simulink model "Mixer"  (R2015a)
settings: Solver=ode2  StartTime=0.0  StopTime=10.0  FixedStep=0.01  RelTol=1e-3
InitFcn:
  | TiltCopter_Parameters_TOSTO_v3
undefined symbols (not defined in the file): Kinv, x1
settings Model: Creator=pela  LastModifiedBy=Claudio
settings HardwareCC: ProdLargestAtomicInteger=Long  ProdLargestAtomicFloat=Double  ProdEndianess=LittleEndian  ProdHWDeviceType=ARM Compatible->ARM Cortex
settings RTWCC: GenCodeOnly=on  GenerateReport=on  Toolchain=Microsoft Visual C++ 2013 v12.0 | nmake (64-bit Windows)  BuildConfiguration=Faster Runs  LaunchReport=on  TargetLang=C++
settings GRTTargetCC: MatFileLogging=off  MultiInstanceERTCode=on  CodeInterfacePackaging=C++ class

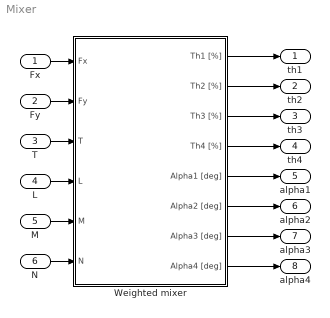
== system Mixer ==
  Fx : Inport
  Fy : Inport  Port=2
  T : Inport  Port=3
  L : Inport  Port=4
  M : Inport  Port=5
  N : Inport  Port=6
  Weighted mixer : Subsystem
  th1 : Outport
  th2 : Outport  Port=2
  th3 : Outport  Port=3
  "th4 " : Outport  Port=4
  alpha1 : Outport  Port=5
  alpha2 : Outport  Port=6
  alpha3 : Outport  Port=7
  alpha4 : Outport  Port=8
  wires:
  T/1 -> Weighted mixer/3(T)
  M/1 -> Weighted mixer/5(M)
  N/1 -> Weighted mixer/6(N)
  Fx/1 -> Weighted mixer/1(Fx)
  Fy/1 -> Weighted mixer/2(Fy)
  L/1 -> Weighted mixer/4(L)
  Weighted mixer/1(Th1 [%]) -> th1/1
  Weighted mixer/2(Th2 [%]) -> th2/1
  Weighted mixer/3(Th3 [%]) -> th3/1
  Weighted mixer/4(Th4 [%]) -> "th4 "/1
  Weighted mixer/5(Alpha1 [deg]) -> alpha1/1
  Weighted mixer/6(Alpha2 [deg]) -> alpha2/1
  Weighted mixer/7(Alpha3 [deg]) -> alpha3/1
  Weighted mixer/8(Alpha4 [deg]) -> alpha4/1

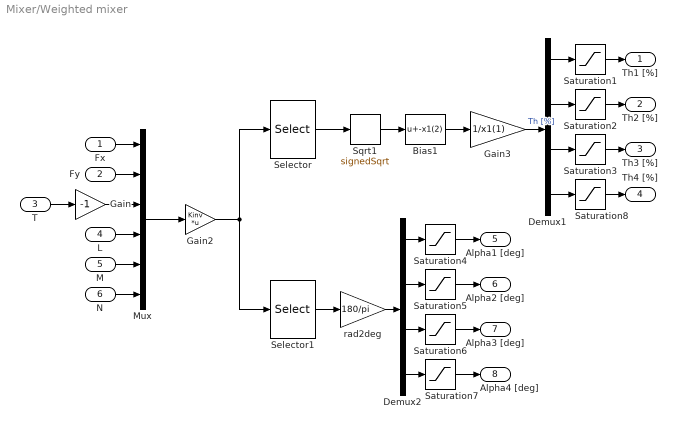
== system Mixer/Weighted mixer ==
  Fx : Inport
  Fy : Inport  Port=2
  T : Inport  Port=3
  L : Inport  Port=4
  M : Inport  Port=5
  N : Inport  Port=6
  Bias1 : Bias  Bias=-x1(2)
  Demux1 : Demux
  Demux2 : Demux
  Gain : Gain  Gain=-1
  Gain2 : Gain  Gain=Kinv  Multiplication=Matrix(K*u)
  Gain3 : Gain  Gain=1/x1(1)
  Mux : Mux  Inputs=6
  Saturation{1..3,8} (4 alike) : Saturate  UpperLimit=100  LowerLimit=0
  Saturation{4..7} (4 alike) : Saturate  UpperLimit=45  LowerLimit=-45
  Selector : Selector  InputPortWidth=8  Indices=[1 2 3 4]
  Selector1 : Selector  InputPortWidth=8  Indices=[5 6 7 8]
  Sqrt1 : Sqrt  Operator=signedSqrt  SaturateOnIntegerOverflow=on
  rad2deg : Gain  Gain=180/pi
  Th1 [%] : Outport
  Th2 [%] : Outport  Port=2
  Th3 [%] : Outport  Port=3
  Th4 [%] : Outport  Port=4
  Alpha1 [deg] : Outport  Port=5
  Alpha2 [deg] : Outport  Port=6
  Alpha3 [deg] : Outport  Port=7
  Alpha4 [deg] : Outport  Port=8
  wires:
  Saturation6/1 -> Alpha3 [deg]/1
  Demux2/1 -> Saturation4/1
  Demux2/3 -> Saturation6/1
  Sqrt1/1 -> Bias1/1
  Bias1/1 -> Gain3/1
  Demux2/2 -> Saturation5/1
  Demux2/4 -> Saturation7/1
  Saturation4/1 -> Alpha1 [deg]/1
  Saturation5/1 -> Alpha2 [deg]/1
  Saturation7/1 -> Alpha4 [deg]/1
  Fx/1 -> Mux/1
  Fy/1 -> Mux/2
  T/1 -> Gain/1
  L/1 -> Mux/4
  M/1 -> Mux/5
  N/1 -> Mux/6
  Selector/1 -> Sqrt1/1
  Selector1/1 -> rad2deg/1
  rad2deg/1 -> Demux2/1
  Gain2/1 -> Selector1/1, Selector/1
  Mux/1 -> Gain2/1
  Demux1/3 -> Saturation3/1
  Demux1/2 -> Saturation2/1
  Demux1/4 -> Saturation8/1
  Demux1/1 -> Saturation1/1
  Saturation1/1 -> Th1 [%]/1
  Saturation2/1 -> Th2 [%]/1
  Saturation3/1 -> Th3 [%]/1
  Saturation8/1 -> Th4 [%]/1
  Gain3/1 -> Demux1/1  "Th [%]"
  Gain/1 -> Mux/3
